simulink model "model_equation"  (R2021a)
settings: Solver=FixedStepAuto  StartTime=0.0  StopTime=10  FixedStep=0.001  RelTol=1e-3
values from neighbouring files (symbols this model uses):
  B_hs = 1e5    (= 100000)    [params.m]
  b_small_bot = 2056.2    [params.m]
  b_small_up = 1350.3    [params.m]
  beta = 0    [params.m]
  bot_damp_start = 0.01054    [params.m]
  C_1 = sqrt(gamma/R*(2/(gamma+1))^((gamma+1)/(gamma-1)))    [params.m]
  C_2 = sqrt((2*gamma)/(R*(gamma-1)))    [params.m]
  C_A_in = 6.6254e-07    [params.m]
  C_A_out = 5.1408e-07    [params.m]
  C_B_in = 5.422e-07    [params.m]
  C_B_out = 1.6346e-06    [params.m]
  flow_C = flow_enable/flow_C_ratio/conv_SI    (= 59999.988)    [params.m]
  flow_C_ratio = dm_max/U_f_max    (= 1)    [params.m]
  flow_noise_var = 1e-10    [params.m]
  g = 9.81    [params.m]
  gamma = 1.4    [params.m]
  gn = 0    [params.m]
  gp = 0.19382    [params.m]
  K_hs = 1e5    (= 100000)    [params.m]
  k_small_bot = 0    [params.m]
  k_small_up = 0    [params.m]
  L = NaN(N,nk)    [hammerstein_wiener_model_estimation.m]    (also in params.m = 0.2)
  lookup_n = [1 2 3 4 5 6 7 8 9 10]    [params.m]
  lookup_q = lookup_q_l*conv_SI*rho    [params.m]
  M = 6.7798462575453    (= 6.77984625755)    [params.m]
  M_L = member.("Settings.Load"){1,1}{1,1}    [identification_faultcode.m]    (also in params.m = 6.25)
  p0 = 1    [params.m]
  p1 = -0.1833    [params.m]
  p2 = 0.0083    [params.m]
  P_0 = 101325    [params.m]
  p_A0 = P_0    (= 101325)    [params.m]
  p_B0 = P_s    (= 600000)    [params.m]
  P_cr = (2/(gamma+1))^(gamma/(gamma-1))    (= 0.528281787717)    [params.m]
  P_s = 6e5    (= 600000)    [params.m]
  prox_bot_band = 4e-4    (= 0.0004)    [params.m]
  prox_up_band = 0.1925    [params.m]
  R = 287.1    [params.m]
  S_0 = S_A-S_B    (= 5.02654824574e-05)    [params.m]
  S_A = (pi*d_A^2)/4    (= 0.000314159265359)    [params.m]
  S_B = S_A-(pi*d_S^2)/4    (= 0.000263893782902)    [params.m]
  SmallDamper_bottom = member.SmallDamper_bottom{1,1}.Variables    [identification_faultcode.m]    (also in params.m = 6)
  SmallDamper_upper = member.SmallDamper_upper{1,1}.Variables    [identification_faultcode.m]    (also in params.m = 4)
  spool_dynamic = 0.012096    [params.m]
  spool_valve_time_delay = 0.020455    [params.m]
  T = cell2mat(T)    [data_driven_models_perfomance.m]    (also in params.m = 281.7)
  Ts = 1e-3    (= 0.001)    [data_driven_models_perfomance.m]    (also in hammerstein_wiener_model_estimation.m; params.m)
  up_damp_start = 0.18123    [params.m]
  V_0A = S_A*0.015    (= 4.71238898038e-06)    [params.m]
  V_0B = S_B*0.015    (= 3.95840674352e-06)    [params.m]
  valve1 = member.ThrottleValve2{1,1}.Variables    [identification_faultcode.m]    (also in params.m = 4)
  valve2 = member.ThrottleValve1{1,1}.Variables    [identification_faultcode.m]    (also in params.m = 2)
libraries: simulink x4
settings Model: OrderedModelArguments=off  Creator=artof  LastModifiedBy=artof
settings SolverCC: AlgebraicLoopSolver=TrustRegion
settings DataIOCC: ExternalInput=[t, u1, u2]  LoadExternalInput=on
settings DebuggingCC: SFMachineParentedDataDiag=warning  UnderSpecifiedDimensionMsg=warning

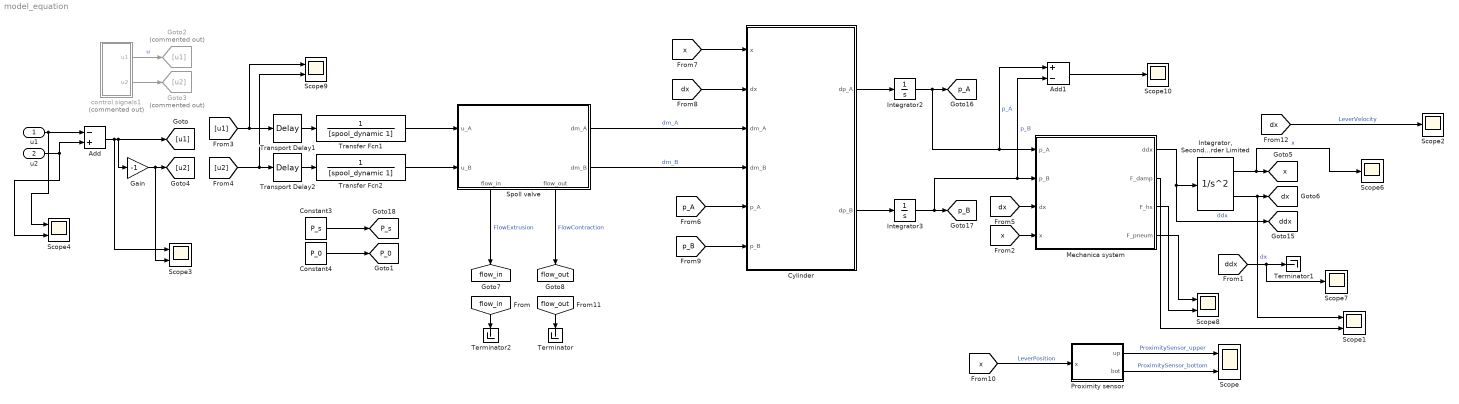
== system model_equation ==
  u1 : Inport
  u2 : Inport  Port=2
  Add : Sum  Inputs=-+
  Add1 : Sum  Inputs=+-
  Constant3 : Constant  Value=P_s
  Constant4 : Constant  Value=P_0
  Cylinder : MATLAB Function  TreatAsAtomicUnit=on
  Gain : Gain  Gain=-1
  Goto2 : Goto  Commented=on  GotoTag=u1
  Goto3 : Goto  Commented=on  GotoTag=u2
  "Integrator, Second-Order Limited" : SecondOrderIntegrator  ICX=x0  LimitX=on  UpperLimitX=gp  LowerLimitX=gn  LimitDXDT=on
  Integrator2 : Integrator  InitialCondition=p_A0
  Integrator3 : Integrator  InitialCondition=p_B0
  Mechanica system : MATLAB Function  TreatAsAtomicUnit=on
  Proximity sensor : MATLAB Function  TreatAsAtomicUnit=on
  Scope{,1,3..4,8..9} (6 alike) : Scope  NumInputPorts=2
  Scope{2,6..7,10} (4 alike) : Scope
  Spoll valve : Subsystem
      settings: PortSchema="{\"entries\":[{\"content\":{\"sides\":[{\"content\":{\"connectorIds\":[\"In1\",\"In2\"]},\"type\":\"ConnectorPlacement.EquallySpacedRectSide\",\"uuid\":\"f49fadee-fa9e-4c00-be17-3013d1757a7f\"},{\"content\":{\"connectorIds\":[\"Out1\",\"Out2\"],\"side\":\"RIGHT\"},\"type\":\"ConnectorPlacement.EquallySpacedRectSide\",\"uuid\":\"640b0073-0df7-45c7-9e72-cb244187d5a1\"},{\"content\":{\"connectorIds\":[],\"side\":\"TOP\"},\"type\":\"ConnectorPlacement.EquallySpacedRectSide\",\"uuid\":\"42e207d6-f026-4ddf-97dc-8c7968fc41f1\"},{\"content\":{\"connectorIds\":[\"Out3\",\"Out4\"],\"side\":\"BOTTOM\"},\"type\":\"ConnectorPlacement.EquallySpacedRectSide\",\"uuid\":\"eeba3cdd-6d70-46a7-a1e2-c2998fe430fd\"}]},\"type\":\"ConnectorPlacement.EquallySpacedConnector\",\"uuid\":\"e8c5a427-dc83-42b8-9540-729b85904a46\"}],\"packageUris\":[\"http://schema.mathworks.com/mf0/Connector/R2020b\"],\"version\":\"1.0\"}"
  Terminator : Terminator
  Terminator1 : Terminator
  Terminator2 : Terminator
  Transfer Fcn1 : TransferFcn  Denominator=[spool_dynamic 1]
  Transfer Fcn2 : TransferFcn  Denominator=[spool_dynamic 1]
  Transport Delay1 : TransportDelay  DelayTime=spool_valve_time_delay
  Transport Delay2 : TransportDelay  DelayTime=spool_valve_time_delay
  control signals1 : Subsystem  Commented=on
  tag scope: P_0=global, P_s=global, ddx=global, dx=global, flow_in=global, flow_out=global, p_A=global, p_B=global, x=global
  wires:
  Mechanica system/1(ddx) -> [ddx], "Integrator, Second-Order Limited"/1  "ddx"
  [ddx] -> Scope7/1, Terminator1/1
  Integrator3/1 -> Add1/2, Mechanica system/2(p_B), [p_B]  "p_B"
  control signals1/2(u2) -> Goto3/1
  Spoll valve/2(dm_B) -> Cylinder/4(dm_B)  "dm_B"
  Spoll valve/1(dm_A) -> Cylinder/3(dm_A)  "dm_A"
  control signals1/1(u1) -> Goto2/1  "u"
  Constant4/1 -> [P_0]
  Cylinder/1(dp_A) -> Integrator2/1
  [x] -> Mechanica system/4(x)
  [p_A] -> Cylinder/5(p_A)
  [x] -> Cylinder/1(x)
  Integrator2/1 -> Add1/1, Mechanica system/1(p_A), [p_A]  "p_A"
  [dx] -> Mechanica system/3(dx)
  [p_B] -> Cylinder/6(p_B)
  Cylinder/2(dp_B) -> Integrator3/1
  Constant3/1 -> [P_s]
  [dx] -> Cylinder/2(dx)
  [u2] -> Scope9/2, Transport Delay2/1
  [u1] -> Scope9/1, Transport Delay1/1
  Transfer Fcn1/1 -> Spoll valve/1(u_A)
  Transfer Fcn2/1 -> Spoll valve/2(u_B)
  Transport Delay1/1 -> Transfer Fcn1/1
  Transport Delay2/1 -> Transfer Fcn2/1
  Proximity sensor/1(up) -> Scope/1  "ProximitySensor_upper"
  Proximity sensor/2(bot) -> Scope/2  "ProximitySensor_bottom"
  "Integrator, Second-Order Limited"/1 -> Scope6/1, [x]  "x"
  "Integrator, Second-Order Limited"/2 -> Scope1/1, [dx]  "dx"
  Spoll valve/4(flow_out) -> [flow_out]  "FlowContraction"
  Spoll valve/3(flow_in) -> [flow_in]  "FlowExtrusion"
  [x] -> Proximity sensor/1(x)  "LeverPosition"
  u1/1 -> Scope4/1, Add/1
  u2/1 -> Scope4/2, Add/2
  Gain/1 -> Scope3/2, [u2]
  [flow_out] -> Terminator/1
  [flow_in] -> Terminator2/1
  Mechanica system/2(F_damp) -> Scope1/2
  [dx] -> Scope2/1  "LeverVelocity"
  Add/1 -> Scope3/1, Gain/1, [u1]
  Mechanica system/4(F_pneum) -> Scope8/1
  Add1/1 -> Scope10/1
  Mechanica system/3(F_hs) -> Scope8/2

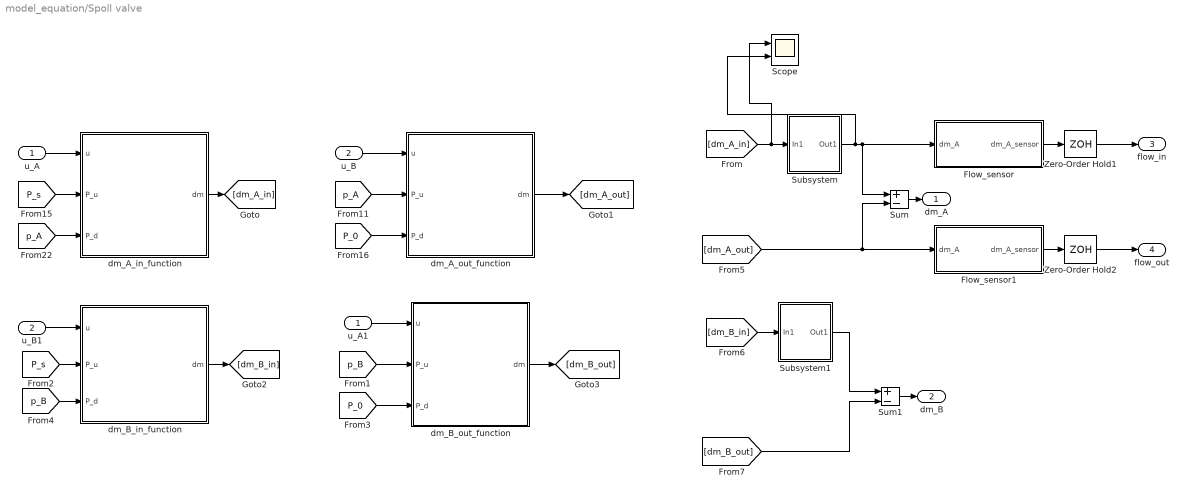
== system model_equation/Spoll valve ==
  u_A : Inport
  u_B : Inport  Port=2
  Flow_sensor : MATLAB Function  TreatAsAtomicUnit=on
  Flow_sensor1 : MATLAB Function  TreatAsAtomicUnit=on
  Scope : Scope  NumInputPorts=2
  Subsystem : Subsystem
  Subsystem1 : Subsystem
  Sum : Sum  Inputs=+-
  Sum1 : Sum  Inputs=+-
  Zero-Order Hold1 : ZeroOrderHold  SampleTime=Ts
  Zero-Order Hold2 : ZeroOrderHold  SampleTime=Ts
  dm_A_in_function : MATLAB Function  TreatAsAtomicUnit=on
  dm_A_out_function : MATLAB Function  TreatAsAtomicUnit=on
  dm_B_in_function : MATLAB Function  TreatAsAtomicUnit=on
  dm_B_out_function : MATLAB Function  TreatAsAtomicUnit=on
  u_A1 : InportShadow
  u_B1 : InportShadow  Port=2
  dm_A : Outport
  dm_B : Outport  Port=2
  flow_in : Outport  Port=3
  flow_out : Outport  Port=4
  wires:
  [P_s] -> dm_A_in_function/2(P_u)
  [p_A] -> dm_A_in_function/3(P_d)
  dm_A_in_function/1(dm) -> [dm_A_in]
  dm_A_out_function/1(dm) -> [dm_A_out]
  [p_A] -> dm_A_out_function/2(P_u)
  [P_0] -> dm_A_out_function/3(P_d)
  u_A/1 -> dm_A_in_function/1(u)
  u_B/1 -> dm_A_out_function/1(u)
  u_B1/1 -> dm_B_in_function/1(u)
  [P_0] -> dm_B_out_function/3(P_d)
  [p_B] -> dm_B_out_function/2(P_u)
  [p_B] -> dm_B_in_function/3(P_d)
  [P_s] -> dm_B_in_function/2(P_u)
  u_A1/1 -> dm_B_out_function/1(u)
  dm_B_in_function/1(dm) -> [dm_B_in]
  dm_B_out_function/1(dm) -> [dm_B_out]
  [dm_A_in] -> Subsystem/1(In1), Scope/1
  Sum/1 -> dm_A/1
  Sum1/1 -> dm_B/1
  [dm_B_out] -> Sum1/2
  [dm_B_in] -> Subsystem1/1(In1)
  Flow_sensor/1(dm_A_sensor) -> Zero-Order Hold1/1
  Flow_sensor1/1(dm_A_sensor) -> Zero-Order Hold2/1
  [dm_A_out] -> Sum/2, Flow_sensor1/1(dm_A)
  Zero-Order Hold1/1 -> flow_in/1
  Zero-Order Hold2/1 -> flow_out/1
  Subsystem1/1(Out1) -> Sum1/1
  Subsystem/1(Out1) -> Scope/2, Sum/1, Flow_sensor/1(dm_A)

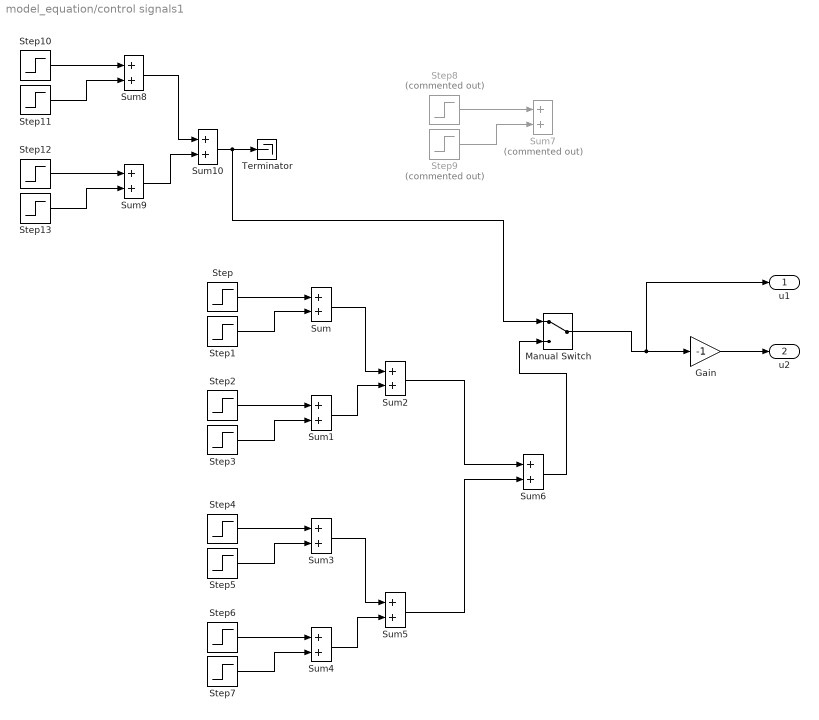
== system model_equation/control signals1 ==
  Gain : Gain  Gain=-1
  Manual Switch : ManualSwitch
  Step : Step  SampleTime=0
  Step1 : Step  Time=1.3  After=-1  SampleTime=0
  Step10 : Step  SampleTime=0
  Step11 : Step  Time=6  After=-1  SampleTime=0
  Step12 : Step  Time=6  After=-1  SampleTime=0
  Step13 : Step  Time=10  SampleTime=0
  Step2 : Step  Time=2  After=-1  SampleTime=0
  Step3 : Step  Time=2.3  SampleTime=0
  Step4 : Step  Time=3  SampleTime=0
  Step5 : Step  Time=3.3  After=-1  SampleTime=0
  Step6 : Step  Time=4  After=-1  SampleTime=0
  Step7 : Step  Time=4.3  SampleTime=0
  Step8 : Step  Commented=on  SampleTime=0
  Step9 : Step  Commented=on  Time=6  After=-1  SampleTime=0
  Sum{,1..6,8..10} (10 alike) : Sum
  Sum7 : Sum  Commented=on
  Terminator : Terminator
  u1 : Outport
  u2 : Outport  Port=2
  wires:
  Gain/1 -> u2/1
  Sum/1 -> Sum2/1
  Step1/1 -> Sum/2
  Step/1 -> Sum/1
  Step3/1 -> Sum1/2
  Step2/1 -> Sum1/1
  Sum1/1 -> Sum2/2
  Sum4/1 -> Sum5/2
  Step6/1 -> Sum4/1
  Step7/1 -> Sum4/2
  Step4/1 -> Sum3/1
  Step5/1 -> Sum3/2
  Sum3/1 -> Sum5/1
  Sum5/1 -> Sum6/2
  Sum2/1 -> Sum6/1
  Sum6/1 -> Manual Switch/2
  Manual Switch/1 -> u1/1, Gain/1
  Step8/1 -> Sum7/1
  Step9/1 -> Sum7/2
  Sum9/1 -> Sum10/2
  Step12/1 -> Sum9/1
  Step13/1 -> Sum9/2
  Step10/1 -> Sum8/1
  Step11/1 -> Sum8/2
  Sum8/1 -> Sum10/1
  Sum10/1 -> Manual Switch/1, Terminator/1

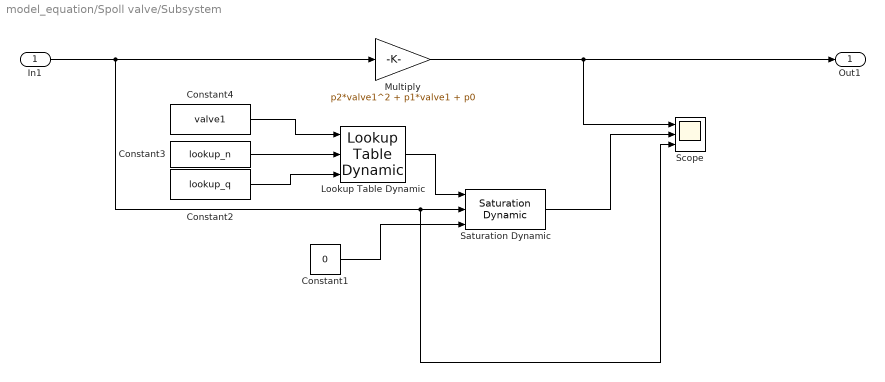
== system model_equation/Spoll valve/Subsystem ==
  In1 : Inport
  Constant1 : Constant  Value=0
  Constant2 : Constant  Value=lookup_q
  Constant3 : Constant  Value=lookup_n
  Constant4 : Constant  Value=valve1
  Lookup Table Dynamic : simulink/Lookup Tables/Lookup Table Dynamic  LookUpMeth=Interpolation-Use End Values  OutDataType=fixdt('double')  OutScaling=[]  OutputDataTypeScalingMode=Specify via dialog  OutDataTypeStr=double  DoSatur=off
  Multiply : Gain  Gain=p2*valve1^2 + p1*valve1 + p0
  Saturation Dynamic : simulink/Discontinuities/Saturation Dynamic  OutMin=[]  OutMax=[]  OutDataTypeStr=Inherit: Same as second input  OutDataType=fixdt(1, 16)  OutScaling=2^-10  DoSatur=off
  Scope : Scope  NumInputPorts=3
  Out1 : Outport
  wires:
  In1/1 -> Scope/3, Saturation Dynamic/2, Multiply/1
  Lookup Table Dynamic/1 -> Saturation Dynamic/1
  Constant2/1 -> Lookup Table Dynamic/3
  Constant3/1 -> Lookup Table Dynamic/2
  Constant4/1 -> Lookup Table Dynamic/1
  Constant1/1 -> Saturation Dynamic/3
  Multiply/1 -> Scope/1, Out1/1
  Saturation Dynamic/1 -> Scope/2

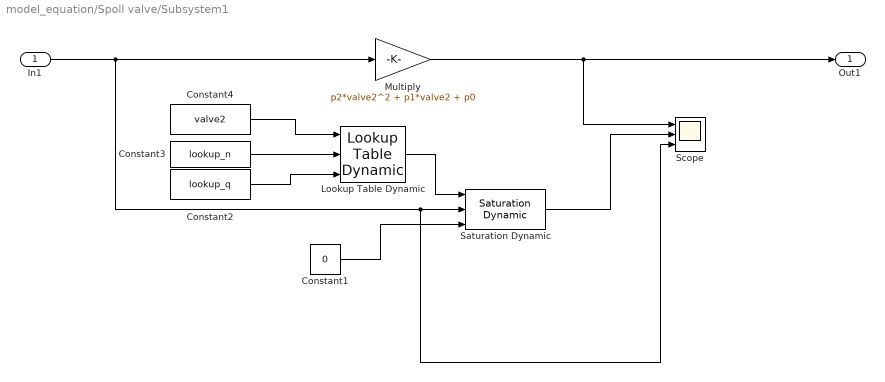
== system model_equation/Spoll valve/Subsystem1 ==
  In1 : Inport
  Constant1 : Constant  Value=0
  Constant2 : Constant  Value=lookup_q
  Constant3 : Constant  Value=lookup_n
  Constant4 : Constant  Value=valve2
  Lookup Table Dynamic : simulink/Lookup Tables/Lookup Table Dynamic  LookUpMeth=Interpolation-Use End Values  OutDataType=fixdt('double')  OutScaling=[]  OutputDataTypeScalingMode=Specify via dialog  OutDataTypeStr=double  DoSatur=off
  Multiply : Gain  Gain=p2*valve2^2 + p1*valve2 + p0
  Saturation Dynamic : simulink/Discontinuities/Saturation Dynamic  OutMin=[]  OutMax=[]  OutDataTypeStr=Inherit: Same as second input  OutDataType=fixdt(1, 16)  OutScaling=2^-10  DoSatur=off
  Scope : Scope  NumInputPorts=3
  Out1 : Outport
  wires:
  Saturation Dynamic/1 -> Scope/2
  Multiply/1 -> Out1/1, Scope/1
  Constant1/1 -> Saturation Dynamic/3
  Constant4/1 -> Lookup Table Dynamic/1
  Constant3/1 -> Lookup Table Dynamic/2
  Constant2/1 -> Lookup Table Dynamic/3
  Lookup Table Dynamic/1 -> Saturation Dynamic/1
  In1/1 -> Multiply/1, Saturation Dynamic/2, Scope/3

== matlab function model_equation/Cylinder ==
  data: x input; dp_A output size=1; dx input; dm_A input; dm_B input; p_A input; p_B input; gamma parameter; V_0A parameter; V_0B parameter; S_A parameter; S_B parameter; R parameter; T parameter; dp_B output size=1; L parameter
function [dp_A,dp_B]= fcn(x,dx,dm_A,dm_B,p_A,p_B,gamma,V_0A,V_0B,S_A,S_B,R,T,L)
V_A = V_0A + S_A*x;
dV_A = dx * S_A;

V_B = V_0B + S_B*(L-x);
dV_B = - dx * S_B;

dp_A = dm_A*gamma*R*T/V_A - p_A*gamma*dV_A/V_A;
dp_B = dm_B*gamma*R*T/V_B - p_B*gamma*dV_B/V_B;
end

== matlab function model_equation/Spoll valve/dm_A_in_function ==
  data: u input; dm output; P_u input; P_d input; C_A_in parameter; C_1 parameter; C_2 parameter; P_cr parameter; T parameter; gamma parameter
function dm = fcn(u, P_u, P_d, C_A_in, C_1, C_2, P_cr, T, gamma)
if u > 0    
    P_ratio = P_d/P_u;
    if P_ratio <= P_cr && P_ratio >= 0
        dm = u*C_A_in*C_1*P_u/sqrt(T);
    elseif P_ratio > P_cr && P_ratio <= 1
        dm = u*C_A_in*C_2*P_u/sqrt(T)*P_ratio^(1/gamma)*sqrt(1-P_ratio^((gamma-1)/gamma));
    else
        %dm = -u*C_A_in*C_2*P_d/sqrt(T)*(1/P_ratio)^(1/gamma)*sqrt(1-(1/P_ratio)^((gamma-1)/gamma));
        dm = 0;
    end
else
    dm = 0;
end

== matlab function model_equation/Spoll valve/dm_A_out_function ==
  data: u input; dm output; P_u input; P_d input; C_A_out parameter; C_1 parameter; P_cr parameter; C_2 parameter; T parameter; gamma parameter
function dm = fcn(u, P_u, P_d, C_A_out, C_1, P_cr, C_2, T, gamma)
if u > 0    
    P_ratio = P_d/P_u;
    if P_ratio <= P_cr && P_ratio >= 0
        dm = u*C_A_out*C_1*P_u/sqrt(T);
    elseif P_ratio > P_cr && P_ratio <= 1
        dm = u*C_A_out*C_2*P_u/sqrt(T)*P_ratio^(1/gamma)*sqrt(1-P_ratio^((gamma-1)/gamma));
    else
        %dm = -u*C_A_out*C_2*P_d/sqrt(T)*(1/P_ratio)^(1/gamma)*sqrt(1-(1/P_ratio)^((gamma-1)/gamma));
        dm = 0;
    end
else
    dm = 0;
end

== matlab function model_equation/Spoll valve/dm_B_in_function ==
  data: u input; dm output; P_u input; P_d input; P_cr parameter; C_B_in parameter; C_1 parameter; C_2 parameter; T parameter; gamma parameter
function dm = fcn(u, P_u, P_d, P_cr, C_B_in, C_1, C_2, T, gamma)
if u > 0    
    P_ratio = P_d/P_u;
    if P_ratio <= P_cr && P_ratio >= 0
        dm = u*C_B_in*C_1*P_u/sqrt(T);
    elseif P_ratio > P_cr && P_ratio <= 1
        dm = u*C_B_in*C_2*P_u/sqrt(T)*P_ratio^(1/gamma)*sqrt(1-P_ratio^((gamma-1)/gamma));
    else
        %dm = -u*C_B_in*C_2*P_d/sqrt(T)*(1/P_ratio)^(1/gamma)*sqrt(1-(1/P_ratio)^((gamma-1)/gamma));
        dm = 0;
    end
else
    dm = 0;
end

== matlab function model_equation/Spoll valve/dm_B_out_function ==
  data: u input; dm output; P_u input; P_d input; P_cr parameter; C_B_out parameter; C_1 parameter; C_2 parameter; T parameter; gamma parameter
function dm = fcn(u, P_u, P_d, P_cr, C_B_out, C_1, C_2, T, gamma)
if u > 0    
    P_ratio = P_d/P_u;
    if P_ratio <= P_cr && P_ratio >= 0
        dm = u*C_B_out*C_1*P_u/sqrt(T);
    elseif P_ratio > P_cr && P_ratio <= 1
        dm = u*C_B_out*C_2*P_u/sqrt(T)*P_ratio^(1/gamma)*sqrt(1-P_ratio^((gamma-1)/gamma));
    else
        %dm = -u*C_B_out*C_2*P_d/sqrt(T)*(1/P_ratio)^(1/gamma)*sqrt(1-(1/P_ratio)^((gamma-1)/gamma));
        dm = 0;
    end
else
    dm = 0;
end

== matlab function model_equation/Proximity sensor ==
  data: x input; up output; bot output; prox_up_band parameter; prox_bot_band parameter
function [up,bot]= fcn(x, prox_up_band, prox_bot_band)
if x >= prox_up_band
    up = 1; bot = 0;
elseif x <= prox_bot_band
    bot = 1; up = 0;
else
    bot = 0;
    up = 0;
end

== matlab function model_equation/Spoll valve/Flow_sensor ==
  settings: updateMethod=DISCRETE
  data: dm_A input; dm_A_sensor output; flow_C parameter; flow_C_ratio parameter; flow_noise_var parameter
function dm_A_sensor = fcn(dm_A, flow_C, flow_C_ratio, flow_noise_var)
dm_A_sensor = flow_C*(flow_C_ratio*dm_A + flow_noise_var*rand());

== matlab function model_equation/Spoll valve/Flow_sensor1 ==
  settings: updateMethod=DISCRETE
  data: dm_A input; dm_A_sensor output; flow_C parameter; flow_C_ratio parameter; flow_noise_var parameter
function dm_A_sensor = fcn(dm_A, flow_C, flow_C_ratio, flow_noise_var)
dm_A_sensor = flow_C*(flow_C_ratio*dm_A + flow_noise_var*rand());

== matlab function model_equation/Mechanica system ==
  data: p_A input; ddx output; p_B input; dx input; x input; S_A parameter; S_B parameter; M parameter; M_L parameter; beta parameter; P_0 parameter; S_0 parameter; g parameter; up_damp_start parameter; bot_damp_start parameter; b_small_up parameter; k_small_up parameter; b_small_bot parameter; k_small_bot parameter; SmallDamper_bottom parameter; SmallDamper_upper parameter; F_damp output; K_hs parameter; B_hs parameter; gp parameter; F_hs output; gn parameter; F_pneum output
function [ddx, F_damp, F_hs, F_pneum] = fcn(p_A, p_B, dx, x, S_A, S_B, M, M_L, beta, P_0, S_0, g, up_damp_start, bot_damp_start, b_small_up, k_small_up, b_small_bot, k_small_bot, SmallDamper_bottom, SmallDamper_upper, K_hs, B_hs, gp, gn)



% % Hard Stop
if 0
up_force = K_hs*(x-gp) + B_hs*dx*ge(dx,0);
bot_force = K_hs*(x-gn) + B_hs*dx*le(dx,0);
% up_force = K_hs*(x-gp) + B_hs*dx*abs(x-gp);
% bot_force = K_hs*(x-gn) + B_hs*dx*abs(x-gn);

% Dead zone calculating Hard Stop
if x >= gp
    F_hs = up_force;
elseif x > gn
    F_hs = 0;
else
    F_hs = bot_force;
end

else
F_hs = 0;
end
% Pneumatic equation
F_pneum = p_A*S_A - p_B*S_B - P_0*S_0;

% Viscous Force
F_beta = dx*beta;

% Dead zone calculating Small Dampers
up_force = k_small_up*(x-up_damp_start) + SmallDamper_upper*b_small_up*dx*ge(dx,0);
bot_force = k_small_bot*(x-bot_damp_start) + SmallDamper_bottom*b_small_bot*dx*le(dx,0);


if x >= up_damp_start
    F_damp = up_force;
elseif x > bot_damp_start
    F_damp = 0;
else
    F_damp = bot_force;
end

% Gravity
F_g = (M + M_L)*g;

% Full mechincal equation
ddx = 1/(M+M_L)*(F_pneum - F_beta - F_hs - F_g - F_damp);
end
